simulink model "TriggeredSubSystem"  (Simulink 7.4)
settings: Solver=ode45  StartTime=0.0  StopTime=10.0  RelTol=1e-3
settings Model: Creator=dread  LastModifiedBy=dread

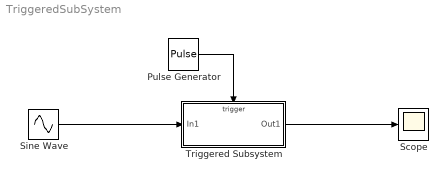
== system TriggeredSubSystem ==
  Pulse Generator : DiscretePulseGenerator  PulseType=Time based  Amplitude=1  Period=1  PulseWidth=5  PhaseDelay=0  SampleTime=1
  Scope : Scope
  Sine Wave : Sin  Amplitude=1  Bias=0  Frequency=1  Phase=0  Samples=10  SampleTime=0  Offset=0
  Triggered Subsystem : Subsystem  TreatAsAtomicUnit=on
  wires:
  Triggered Subsystem/1(Out1) -> Scope/1
  Sine Wave/1 -> Triggered Subsystem/1(In1)
  Pulse Generator/1 -> Triggered Subsystem/Trigger

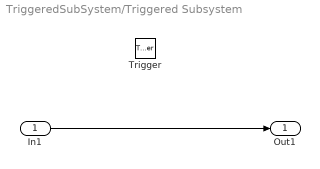
== system TriggeredSubSystem/Triggered Subsystem ==
  In1 : Inport  OutDataType=fixdt(1, 16)  OutScaling=2^0
  Trigger : TriggerPort  TriggerType=either
  Out1 : Outport  OutDataType=fixdt(1, 16)  OutScaling=2^0
  wires:
  In1/1 -> Out1/1
